simulink model "untitled"  (R2018b)
settings: Solver=VariableStepAuto  StartTime=0.0  StopTime=5  RelTol=1e-3
libraries: commsynccomp2 x1
settings Model: Creator=nhat  LastModifiedBy=nhat

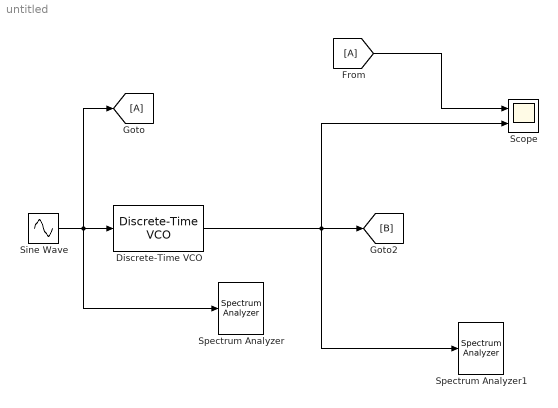
== system untitled ==
  Discrete-Time VCO : commsynccomp2/Discrete-Time VCO  Ac=5  Fc=3000  Kc=2000  Ph=0  ts=1/20000
      settings: SourceProductName=Communications System Toolbox  SourceProductBaseCode=CM
  Scope : Scope  NumInputPorts=2
  Sine Wave : Sin  Frequency=500*2*pi  SampleTime=1/20000
  Spectrum Analyzer : SpectrumAnalyzer
  Spectrum Analyzer1 : SpectrumAnalyzer
  wires:
  Sine Wave/1 -> Spectrum Analyzer/1, [A], Discrete-Time VCO/1
  Discrete-Time VCO/1 -> Scope/2, Spectrum Analyzer1/1, [B]
  [A] -> Scope/1
